simulink model "DC_Motor_SC"  (Simulink 10.3)
settings: Solver=ode45  StartTime=0.0  StopTime=30  FixedStep=1e-2  RelTol=1e-3  EnableMultiTasking=on
undefined symbols (not defined in the file): Kd, Ki, Kp
settings Model: Creator=kiran.kulkarni  LastModifiedBy=Yogesh  MultithreadedSim=on
settings DataIOCC: LimitDataPoints=on
settings OptimizationCC: InitFltsAndDblsToZero=on
settings DebuggingCC: SaveWithParameterizedLinksMsg=none  SignalResolutionControl=TryResolveAllWithWarning  SolverPrmCheckMsg=warning  MultiTaskDSMMsg=warning  MultiTaskCondExecSysMsg=none
settings GRTTargetCC: TargetFcnLib=ansi_tfl_tmw.mat

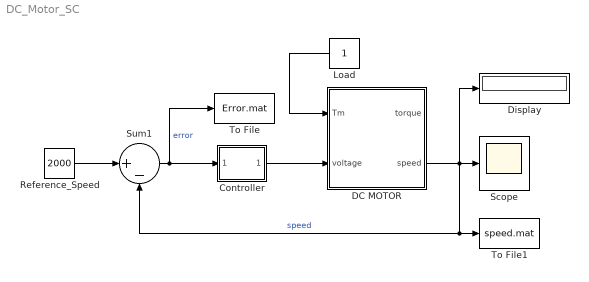
== system DC_Motor_SC ==
  Controller : Subsystem  mask(PID Controller){P=Kp, I=Ki, D=Kd}
      mask prompts: P "Proportional:"; I "Integral"; D "Derivative:"
      mask help: Enter expressions for proportional, integral, and derivative terms.
      mask Help: This block implements a PID controller where paramaters are entered for the Proportional, Integral and Derivative terms.
      mask Display: disp('PID')
  DC MOTOR : Subsystem
  Display : Display
  Load : Constant
  Reference_Speed : Constant  Value=2000
  Scope : Scope
  Sum1 : Sum  Inputs=|+-
  To File : ToFile  Filename=Error.mat  MatrixName=Error
  To File1 : ToFile  Filename=speed.mat  MatrixName=speed
  wires:
  DC MOTOR/2(speed) -> Display/1, Sum1/2, To File1/1, Scope/1  "speed"
  Load/1 -> DC MOTOR/1(Tm)
  Reference_Speed/1 -> Sum1/1
  Sum1/1 -> Controller/1(In_1), To File/1  "error"
  Controller/1(Out_1) -> DC MOTOR/2(voltage)

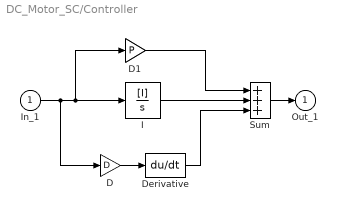
== system DC_Motor_SC/Controller ==
  In_1 : Inport
  D : Gain  Gain=D  SaturateOnIntegerOverflow=on  OutDataTypeStr=Inherit: Same as input  ParamDataTypeStr=Inherit: Same as input
  D1 : Gain  Gain=P  SaturateOnIntegerOverflow=on  OutDataTypeStr=Inherit: Same as input  ParamDataTypeStr=Inherit: Same as input
  Derivative : Derivative
  I : TransferFcn  Numerator=[I]  Denominator=[1 0]
  Sum : Sum  Inputs=+++  InputSameDT=on  SaturateOnIntegerOverflow=on  OutDataTypeStr=Inherit: Same as first input
  Out_1 : Outport  InitialOutput=0  VectorParamsAs1DForOutWhenUnconnected=off
  wires:
  D1/1 -> Sum/1
  I/1 -> Sum/2
  Derivative/1 -> Sum/3
  D/1 -> Derivative/1
  Sum/1 -> Out_1/1
  In_1/1 -> D/1, I/1, D1/1

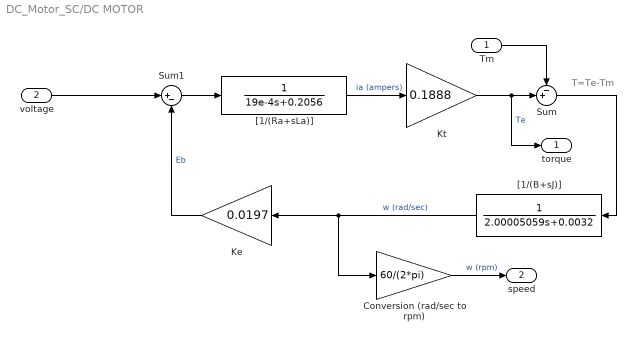
== system DC_Motor_SC/DC MOTOR ==
  note: T=Te-Tm
  Tm : Inport
  voltage : Inport  Port=2
  Conversion (rad/sec to rpm) : Gain  Gain=60/(2*pi)
  Ke : Gain  Gain=0.0197
  Kt : Gain  Gain=0.1888
  Sum : Sum  Inputs=-+|
  Sum1 : Sum  Inputs=|+-
  "[1/(B+sJ)]" : TransferFcn  Numerator=1  Denominator=[2.00005059 0.0032]
  "[1/(Ra+sLa)]" : TransferFcn  Numerator=1  Denominator=[19e-4 0.2056]
  torque : Outport  VectorParamsAs1DForOutWhenUnconnected=off
  speed : Outport  Port=2  VectorParamsAs1DForOutWhenUnconnected=off
  wires:
  Sum1/1 -> "[1/(Ra+sLa)]"/1
  Ke/1 -> Sum1/2  "Eb"
  Kt/1 -> torque/1, Sum/2  "Te"
  Sum/1 -> "[1/(B+sJ)]"/1
  "[1/(Ra+sLa)]"/1 -> Kt/1  "ia (ampers)"
  voltage/1 -> Sum1/1
  Tm/1 -> Sum/1
  "[1/(B+sJ)]"/1 -> Ke/1, Conversion (rad/sec to rpm)/1  "w (rad/sec)"
  Conversion (rad/sec to rpm)/1 -> speed/1  "w (rpm)"
